simulink model "Lab1A_C1"  (R2019b)
settings: Solver=ode45  StartTime=0.0  StopTime=3  RelTol=1e-3  AbsTol=1e-6
settings Model: Creator=sinow  LastModifiedBy=sinow

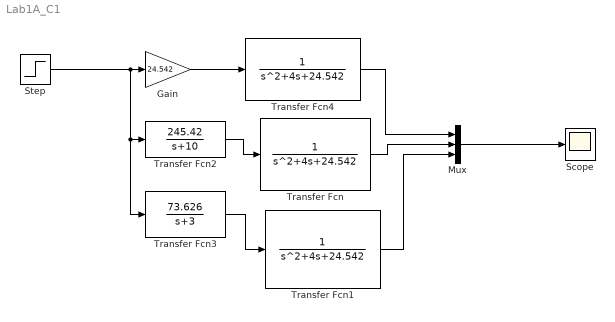
== system Lab1A_C1 ==
  Gain : Gain  Gain=24.542
  Mux : Mux  Inputs=3
  Scope : Scope
  Step : Step  Time=0  SampleTime=0
  Transfer Fcn : TransferFcn  Denominator=[1 4 24.542]
  Transfer Fcn1 : TransferFcn  Denominator=[1 4 24.542]
  Transfer Fcn2 : TransferFcn  Numerator=[245.42]  Denominator=[1 10]
  Transfer Fcn3 : TransferFcn  Numerator=[73.626]  Denominator=[1 3]
  Transfer Fcn4 : TransferFcn  Numerator=1  Denominator=[1 4 24.542]
  wires:
  Step/1 -> Transfer Fcn3/1, Transfer Fcn2/1, Gain/1
  Gain/1 -> Transfer Fcn4/1
  Transfer Fcn2/1 -> Transfer Fcn/1
  Transfer Fcn3/1 -> Transfer Fcn1/1
  Transfer Fcn/1 -> Mux/2
  Transfer Fcn1/1 -> Mux/3
  Transfer Fcn4/1 -> Mux/1
  Mux/1 -> Scope/1
